simulink model "torch_xdof_sim"  (R2025b)
settings: Solver=VariableStepAuto  StartTime=0.0  StopTime=120  RelTol=1e-3
values from neighbouring files (symbols this model uses):
  framePeriod_s = 1/frameRate_hz    (= 0.005)    [setup.m]
  frameRate_hz = 200    [setup.m]
  initial_position = cur_x(1)/100    [sim_vs_flight.m]    (also in untitled2.m = -1*cur_z(1))
undefined symbols (not defined in the file or in its folder): Aircraft, magnitude
libraries: simulink x19, slpidlib x4, simulink_extras x3, uavutilslib x1, dspmathops x1
(part 1 of 2)
settings Model: Creator=amark  LastModifiedBy=aerol

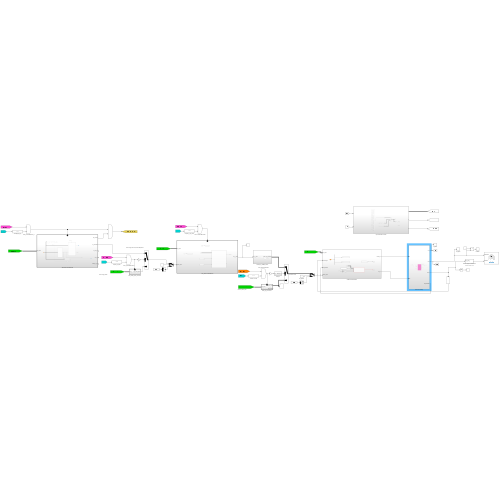
[thumbnail: Simulink's stored preview of the top-level diagram]
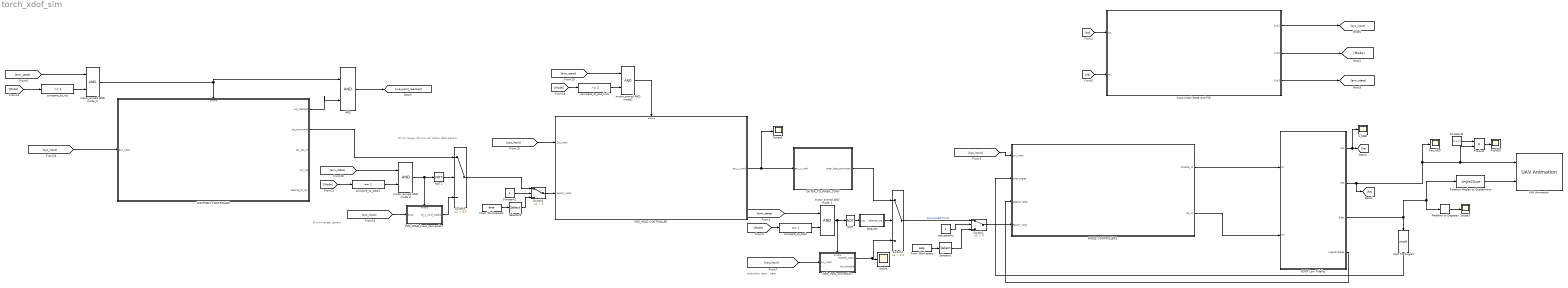
== system torch_xdof_sim ==
  note: telemetry data . para
  note: tf mini range, param
  note: tfmini range, bfs ins vel, telem data param
  6DOF Low Fidelity : Subsystem
  AND : Logic  IconShape=distinctive  AllPortsSameDT=off  OutDataTypeStr=boolean
  ANGLE CONTROLLER1 : Subsystem
  Cast To Single1 : DataTypeConversion  OutDataTypeStr=single  SaturateOnIntegerOverflow=off  RndMeth=Floor
  Constant1 : Constant
  Constant4 : Constant  Value=[1,1,-1]
  From Workspace : FromWorkspace  VariableName=data  SampleTime=0.005
  From Workspace1 : FromWorkspace  VariableName=data  OutDataTypeStr=double  SampleTime=0.005
  Input Initial State and PID : Subsystem
  NOT : Logic  Operator=NOT  IconShape=distinctive  AllPortsSameDT=off  OutDataTypeStr=boolean
  NOT1 : Logic  Operator=NOT  IconShape=distinctive  AllPortsSameDT=off  OutDataTypeStr=boolean
  OUTER_TO_INNER_CONV : Subsystem
  POS_HOLD CONTROLLER : Subsystem
  POS_HOLD_input_conversion : Subsystem
  PosNEU : Scope
      settings: ActiveDisplayYMinimum=-0.14999999999999997  ActiveDisplayYMaximum=1.3499999999999999
  Pos_NED : Scope
      settings: ActiveDisplayYMinimum=-13.68929465533385  ActiveDisplayYMaximum=21.935482841830105  DataLoggingVariableName=ScopeData7
  Product : Product
  Radians to Degrees : simulink_extras/Transformations/Radians to Degrees
  Rotation Angles to Quaternions : Angle2Quat  rotationOrder=XYZ
      settings: AttributesFormatString=Rotation Order: %<rotationOrder>
  Scope : Scope
      settings: DataLoggingVariableName=ScopeData5
  Scope1 : Scope
      settings: ActiveDisplayYMinimum=-1  ActiveDisplayYMaximum=1  DataLoggingVariableName=ScopeData8
  Scope3 : Scope
      settings: ActiveDisplayYMinimum=-18.742986936261055  ActiveDisplayYMaximum=18.74922049710748  DataLoggingVariableName=ScopeData3
  Selector1 : Selector  InputPortWidth=4  IndexOptions=Index vector (dialog)  Indices=[1 2]  OutputSizes=1
  Selector2 : Selector  InputPortWidth=4  IndexOptions=Index vector (dialog)  Indices=3  OutputSizes=1
  Stab_input_conversion : Subsystem
  Switch1 : Switch  Criteria=u2 > Threshold  SaturateOnIntegerOverflow=off  InputSameDT=off
  Switch2 : Switch  Criteria=u2 > Threshold  Threshold=0.5  SaturateOnIntegerOverflow=off  InputSameDT=off
  Switch3 : Switch  Criteria=u2 > Threshold  Threshold=0.5  SaturateOnIntegerOverflow=off  InputSameDT=off
  Switch4 : Switch  Criteria=u2 > Threshold  SaturateOnIntegerOverflow=off  InputSameDT=off
  UAV Animation : uavutilslib/UAV Animation  NumUAV=1  DynamicUAVConfig=off  UAVType=Multirotor  UAVSize=1  UAVColor=[1 0 0]  UAVTrajectoryAlpha=1  InertialZDirection=Down  RotationFormat=Quaternion  DrawMarkers=off  SampleTime=0.5
  V_NED : Scope
      settings: ActiveDisplayYMinimum=-0.14995297580074798  ActiveDisplayYMaximum=1.3495767822067306  DataLoggingVariableName=ScopeData2
  WAYPOINT CONTROLLER : Subsystem
  compare_to_pos_hold : simulink/Logic and Bit Operations/Compare To Constant  relop=>=  const=2  OutDataTypeStr=boolean
  compare_to_stab : simulink/Logic and Bit Operations/Compare To Constant  relop===  const=1  OutDataTypeStr=boolean
  compare_to_stab1 : simulink/Logic and Bit Operations/Compare To Constant  relop===  const=2  OutDataTypeStr=boolean
  compare_to_wp : simulink/Logic and Bit Operations/Compare To Constant  relop=>=  const=3  OutDataTypeStr=boolean
  delayed : Subsystem
  motor_armed AND mode 1 : Logic  IconShape=distinctive  AllPortsSameDT=off  OutDataTypeStr=boolean
  motor_armed AND mode 2 : Logic  IconShape=distinctive  AllPortsSameDT=off  OutDataTypeStr=boolean
  motor_armed AND mode2 : Logic  IconShape=distinctive  AllPortsSameDT=off  OutDataTypeStr=boolean
  motor_armed AND mode_3 : Logic  IconShape=distinctive  AllPortsSameDT=off  OutDataTypeStr=boolean
  use_params : Constant
  wires:
  ANGLE CONTROLLER1/2(roll_cc) -> 6DOF Low Fidelity/2(Mx)
  6DOF Low Fidelity/3(Euler) -> Cast To Single1/1, Rotation Angles to Quaternions/1, Radians to Degrees/1
  POS_HOLD CONTROLLER/1(acc_y_cmd) -> Scope1/1, OUTER_TO_INNER_CONV/1(acc_y_cmd)
  Cast To Single1/1 -> ANGLE CONTROLLER1/2(euler angles)
  Constant4/1 -> Product/1
  Product/1 -> PosNEU/1
  ANGLE CONTROLLER1/1(throttle_cc) -> 6DOF Low Fidelity/1(Fz)
  Rotation Angles to Quaternions/1 -> UAV Animation/2
  [Xe] -> Input Initial State and PID/1(In1)
  Input Initial State and PID/1(Out1) -> [sys_input]
  Input Initial State and PID/3(Out3) -> [arm_state]
  Input Initial State and PID/2(Out2) -> [Mode]
  [Ve] -> Input Initial State and PID/2(In2)
  6DOF Low Fidelity/2(Xe1) -> [Xe], UAV Animation/1, Product/2, Pos_NED/1
  6DOF Low Fidelity/1(Ve1) -> V_NED/1, [Ve]
  6DOF Low Fidelity/4(Angular Rates) -> ANGLE CONTROLLER1/3(angular rates)
  [sys_input] -> ANGLE CONTROLLER1/1(sys_input)
  use_params/1 -> Switch1/2
  From Workspace/1 -> Selector1/1
  Selector1/1 -> Switch1/3
  Switch1/1 -> ANGLE CONTROLLER1/4(Param_input)
  motor_armed AND mode 1/1 -> NOT/1, Stab_input_conversion/Enable
  Stab_input_conversion/1(throttle_input) -> Scope/1, Switch2/3
  NOT/1 -> delayed/1(sig)
  compare_to_stab/1 -> motor_armed AND mode 1/2
  [sys_input] -> Stab_input_conversion/1(sys_input)
  [arm_state] -> motor_armed AND mode 1/1
  [Mode] -> compare_to_stab/1
  OUTER_TO_INNER_CONV/1(inner_loop_command) -> Switch2/1
  delayed/1(delayed_sig) -> Switch2/2
  Switch2/1 -> Switch1/1  "Commanded Thrust"
  [Mode] -> compare_to_pos_hold/1
  [arm_state] -> motor_armed AND mode2/1
  motor_armed AND mode2/1 -> POS_HOLD CONTROLLER/Enable
  compare_to_pos_hold/1 -> motor_armed AND mode2/2
  motor_armed AND mode 2/1 -> NOT1/1, POS_HOLD_input_conversion/Enable
  compare_to_stab1/1 -> motor_armed AND mode 2/2
  [arm_state] -> motor_armed AND mode 2/1
  [sys_input] -> POS_HOLD_input_conversion/1(Sys1)
  [Mode] -> compare_to_stab1/1
  POS_HOLD_input_conversion/1(ve_z_cmd_input1) -> Switch3/3
  From Workspace1/1 -> Selector2/1
  NOT1/1 -> Switch3/2
  Selector2/1 -> Switch4/3
  Switch3/1 -> Switch4/1
  Constant1/1 -> Switch4/2
  Switch4/1 -> POS_HOLD CONTROLLER/2(param_input)
  [sys_input] -> POS_HOLD CONTROLLER/1(Sys_input)
  [sys_input] -> WAYPOINT CONTROLLER/1(Sys_input)
  [arm_state] -> motor_armed AND mode_3/1
  compare_to_wp/1 -> motor_armed AND mode_3/2
  [Mode] -> compare_to_wp/1
  motor_armed AND mode_3/1 -> WAYPOINT CONTROLLER/Enable, AND/1
  WAYPOINT CONTROLLER/1(wp_reached) -> AND/2
  AND/1 -> [waypoint_reached]
  WAYPOINT CONTROLLER/2(wp_command) -> Switch3/1
  Radians to Degrees/1 -> Scope3/1

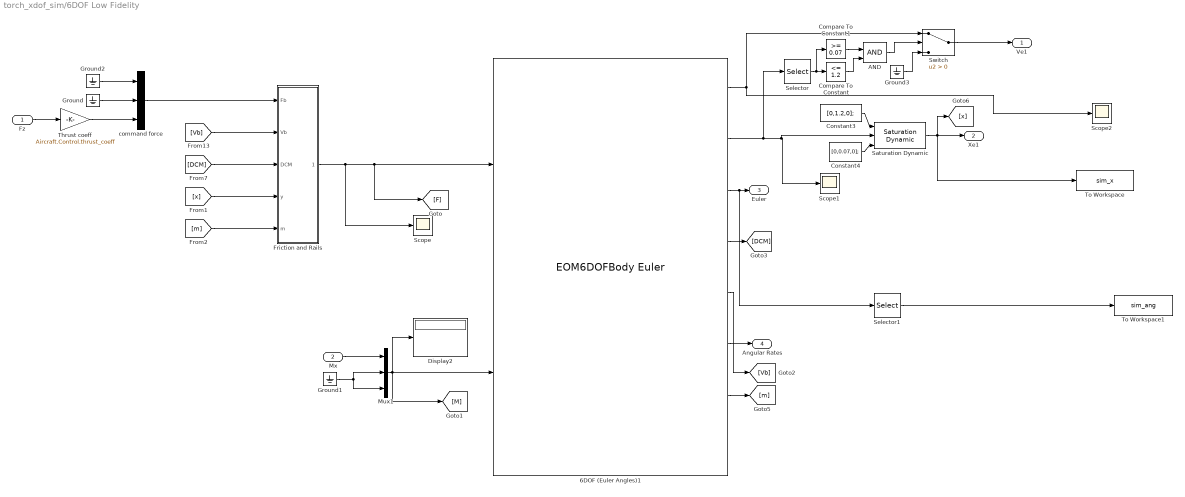
== system torch_xdof_sim/6DOF Low Fidelity ==
  Fz : Inport
  Mx : Inport  Port=2
  6DOF (Euler Angles)1 : EOM6DOFBodyEuler  xme_0=[0 initial_position 0]  mass_0=Aircraft.Mass.mass_kg  inertia=diag([3.2e-4,1e-20,1e-20])  mass_flag=on
  AND : Logic  IconShape=distinctive  AllPortsSameDT=off  OutDataTypeStr=boolean
  Compare To Constant : simulink/Logic and Bit Operations/Compare To Constant  relop=<=  const=1.2  OutDataTypeStr=boolean
  Compare To Constant1 : simulink/Logic and Bit Operations/Compare To Constant  relop=>=  const=0.07  OutDataTypeStr=boolean
  Constant3 : Constant  Value=[0,1.2,0];
  Constant4 : Constant  Value=[0,0.07,0];
  Display2 : Display
  Friction and Rails : MATLAB Function  TreatAsAtomicUnit=on
  Ground{,1..3} (4 alike) : Ground
  Mux1 : Mux  Inputs=3
  Saturation Dynamic : simulink/Discontinuities/Saturation Dynamic  OutMin=[]  OutMax=[]  OutDataTypeStr=Inherit: Same as second input  OutDataType=fixdt(1, 16)  OutScaling=2^-10  DoSatur=off
  Scope : Scope
      settings: ActiveDisplayYMinimum=-0.077435500148142641  ActiveDisplayYMaximum=0.69691950133328384  DataLoggingVariableName=ScopeData4
  Scope1 : Scope
      settings: ActiveDisplayYMinimum=-1  ActiveDisplayYMaximum=1
  Scope2 : Scope
      settings: ActiveDisplayYMinimum=-1  ActiveDisplayYMaximum=1  DataLoggingVariableName=ScopeData6
  Selector : Selector  InputPortWidth=3  IndexOptions=Index vector (dialog)  Indices=[2]  OutputSizes=1
  Selector1 : Selector  InputPortWidth=3  IndexOptions=Index vector (dialog)  Indices=1  OutputSizes=1
  Switch : Switch  Criteria=u2 > Threshold  SaturateOnIntegerOverflow=off  InputSameDT=off
  Thrust coeff : Gain  Gain=Aircraft.Control.thrust_coeff
  To Workspace : ToWorkspace  VariableName=sim_x  SaveFormat=Timeseries  SampleTime=-1
  To Workspace1 : ToWorkspace  VariableName=sim_ang  SaveFormat=Timeseries  SampleTime=-1
  command force : Mux  Inputs=3
  Ve1 : Outport
  Xe1 : Outport  Port=2
  Euler : Outport  Port=3
  Angular Rates : Outport  Port=4
  wires:
  Mux1/1 -> 6DOF (Euler Angles)1/2, [M], Display2/1
  6DOF (Euler Angles)1/3 -> Selector1/1, Euler/1
  Mx/1 -> Mux1/1
  command force/1 -> Friction and Rails/1(Fb)
  Ground1/1 -> Mux1/3, Mux1/2
  6DOF (Euler Angles)1/5 -> [Vb]
  Ground2/1 -> command force/1
  Fz/1 -> Thrust coeff/1
  6DOF (Euler Angles)1/4 -> [DCM]
  [DCM] -> Friction and Rails/3(DCM)
  [Vb] -> Friction and Rails/2(Vb)
  Ground/1 -> command force/2
  Thrust coeff/1 -> command force/3
  Friction and Rails/1(output) -> Scope/1, [F], 6DOF (Euler Angles)1/1
  [x] -> Friction and Rails/4(y)
  6DOF (Euler Angles)1/7 -> [m]
  [m] -> Friction and Rails/5(m)
  Compare To Constant1/1 -> AND/1
  Selector/1 -> Compare To Constant1/1, Compare To Constant/1
  AND/1 -> Switch/2
  Ground3/1 -> Switch/3
  Compare To Constant/1 -> AND/2
  Constant4/1 -> Saturation Dynamic/3
  Constant3/1 -> Saturation Dynamic/1
  6DOF (Euler Angles)1/2 -> Saturation Dynamic/2, Scope1/1, Selector/1
  6DOF (Euler Angles)1/1 -> Scope2/1, Switch/1
  Saturation Dynamic/1 -> To Workspace/1, Xe1/1, [x]
  Switch/1 -> Ve1/1
  6DOF (Euler Angles)1/6 -> Angular Rates/1
  Selector1/1 -> To Workspace1/1

== system torch_xdof_sim/ANGLE CONTROLLER1 ==
  sys_input : Inport
  euler angles : Inport  Port=2
  angular rates : Inport  Port=3
  Param_input : Inport  Port=4
  Demux : Demux  Outputs=3
  Demux1 : Demux  Outputs=2
  Roll Controller : Subsystem
  throttle_cc : Outport
  roll_cc : Outport  Port=2
  wires:
  Roll Controller/1(roll_cc) -> roll_cc/1  "roll_cc"
  [throttle_cc] -> throttle_cc/1  "throttle"
  euler angles/1 -> Demux/1
  Demux/1 -> Roll Controller/3(roll_angle_rad)  "roll_angle"
  angular rates/1 -> Roll Controller/4(roll_rate_radps)
  [roll_angle_cmd_rad] -> Roll Controller/2(Roll_angle_cmd_rad)  "roll_cmd"
  sys_input/1 -> Roll Controller/1(sys_input)
  Demux1/2 -> [roll_angle_cmd_rad]
  Param_input/1 -> Demux1/1
  Demux1/1 -> [throttle_cc]

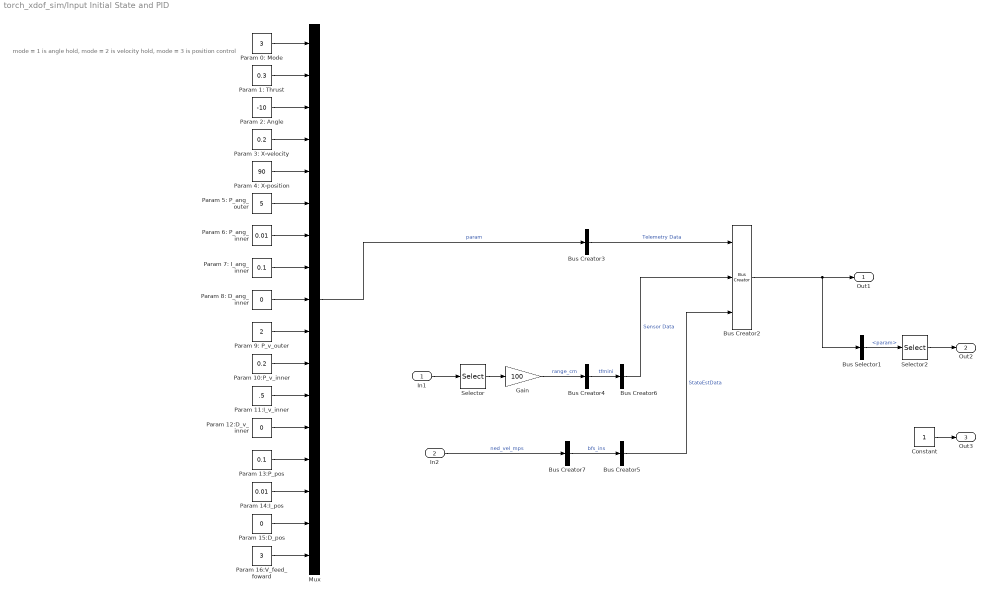
== system torch_xdof_sim/Input Initial State and PID ==
  note: mode = 1 is angle hold, mode = 2 is velocity hold, mode = 3 is position control
  In1 : Inport
  In2 : Inport  Port=2
  Bus Creator2 : BusCreator  Inputs=3
  Bus Creator{3..7} (5 alike) : BusCreator  Inputs=1
  Bus Selector1 : BusSelector  OutputSignals=Telemetry Data.param
  Constant : Constant
  Gain : Gain  Gain=100
  Mux : Mux  Inputs=17
  Param 0: Mode : Constant  Value=3
  Param 10:P_v_inner : Constant  Value=0.2
  Param 11:I_v_inner : Constant  Value=.5
  Param 12:D_v_inner : Constant  Value=0
  Param 13:P_pos : Constant  Value=0.1
  Param 14:I_pos : Constant  Value=0.01
  Param 15:D_pos : Constant  Value=0
  Param 16:V_feed_foward : Constant  Value=3
  Param 1: Thrust : Constant  Value=0.3
  Param 2: Angle : Constant  Value=-10
  Param 3: X-velocity : Constant  Value=0.2
  Param 4: X-position : Constant  Value=90
  Param 5: P_ang_outer : Constant  Value=5
  Param 6: P_ang_inner : Constant  Value=0.01
  Param 7: I_ang_inner : Constant  Value=0.1
  Param 8: D_ang_inner : Constant  Value=0
  Param 9: P_v_outer : Constant  Value=2
  Selector : Selector  InputPortWidth=3  IndexOptions=Index vector (dialog)  Indices=2  OutputSizes=1
  Selector2 : Selector  IndexMode=Zero-based  InputPortWidth=17  IndexOptions=Index vector (dialog)  Indices=0  OutputSizes=1
  Out1 : Outport
  Out2 : Outport  Port=2
  Out3 : Outport  Port=3
  wires:
  Param 3: X-velocity/1 -> Mux/4
  Bus Creator5/1 -> Bus Creator2/3  "StateEstData"
  Param 2: Angle/1 -> Mux/3
  Param 4: X-position/1 -> Mux/5
  Selector/1 -> Gain/1
  Param 11:I_v_inner/1 -> Mux/12
  Param 10:P_v_inner/1 -> Mux/11
  Param 9: P_v_outer/1 -> Mux/10
  Bus Creator6/1 -> Bus Creator2/2  "Sensor Data"
  Param 7: I_ang_inner/1 -> Mux/8
  Param 1: Thrust/1 -> Mux/2
  Param 5: P_ang_outer/1 -> Mux/6
  Bus Creator4/1 -> Bus Creator6/1  "tfmini"
  Bus Creator3/1 -> Bus Creator2/1  "Telemetry Data"
  Param 8: D_ang_inner/1 -> Mux/9
  Param 0: Mode/1 -> Mux/1
  Gain/1 -> Bus Creator4/1  "range_cm"
  Param 6: P_ang_inner/1 -> Mux/7
  In1/1 -> Selector/1
  In2/1 -> Bus Creator7/1  "ned_vel_mps"
  Bus Creator7/1 -> Bus Creator5/1  "bfs_ins"
  Bus Selector1/1 -> Selector2/1  "<param>"
  Bus Creator2/1 -> Bus Selector1/1, Out1/1
  Selector2/1 -> Out2/1
  Constant/1 -> Out3/1
  Mux/1 -> Bus Creator3/1  "param"
  Param 16:V_feed_foward/1 -> Mux/17
  Param 12:D_v_inner/1 -> Mux/13
  Param 13:P_pos/1 -> Mux/14
  Param 14:I_pos/1 -> Mux/15
  Param 15:D_pos/1 -> Mux/16

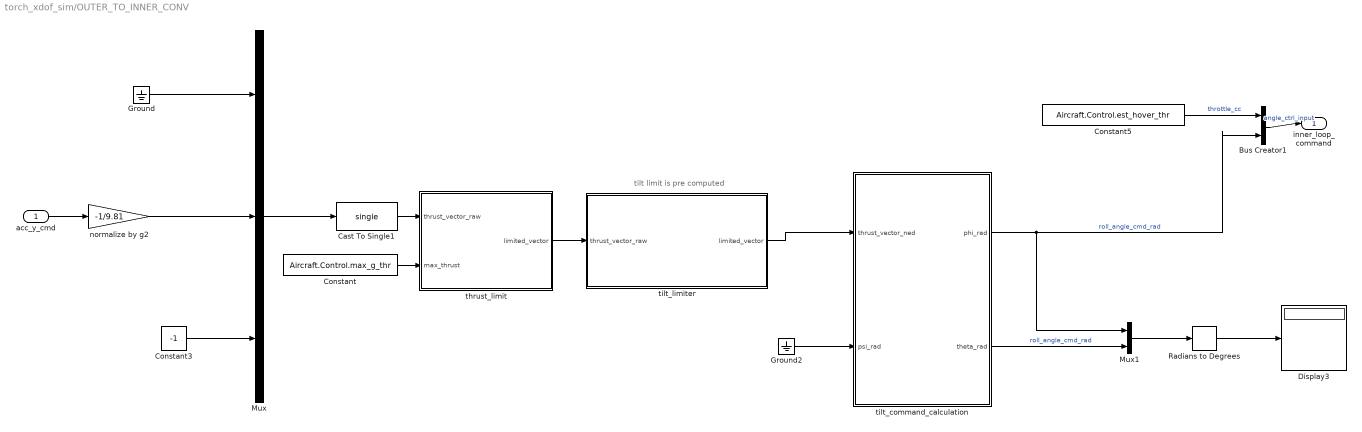
== system torch_xdof_sim/OUTER_TO_INNER_CONV ==
  note: tilt limit is pre computed
  acc_y_cmd : Inport
  " tilt_limiter" : MATLAB Function  TreatAsAtomicUnit=on
  Bus Creator1 : BusCreator  Inputs=2
  Cast To Single1 : DataTypeConversion  OutDataTypeStr=single  SaturateOnIntegerOverflow=off  RndMeth=Floor
  Constant : Constant  Value=Aircraft.Control.max_g_thr  OutDataTypeStr=single
  Constant3 : Constant  Value=-1
  Constant5 : Constant  Value=Aircraft.Control.est_hover_thr  OutDataTypeStr=single
  Display3 : Display
  Ground : Ground
  Ground2 : Ground
  Mux : Mux  Inputs=3
  Mux1 : Mux  Inputs=2
  Radians to Degrees : simulink_extras/Transformations/Radians to Degrees
  normalize by g2 : Gain  Gain=-1/9.81
  thrust_limit : MATLAB Function  TreatAsAtomicUnit=on
  tilt_command_calculation : MATLAB Function  TreatAsAtomicUnit=on
  inner_loop_command : Outport
  wires:
  Constant/1 -> thrust_limit/2(max_thrust)
  thrust_limit/1(limited_vector) -> " tilt_limiter"/1(thrust_vector_raw)
  " tilt_limiter"/1(limited_vector) -> tilt_command_calculation/1(thrust_vector_ned)
  tilt_command_calculation/1(phi_rad) -> Bus Creator1/2, Mux1/1  "roll_angle_cmd_rad"
  tilt_command_calculation/2(theta_rad) -> Mux1/2  "roll_angle_cmd_rad"
  Constant5/1 -> Bus Creator1/1  "throttle_cc"
  Ground/1 -> Mux/1
  normalize by g2/1 -> Mux/2
  Ground2/1 -> tilt_command_calculation/2(psi_rad)
  Mux/1 -> Cast To Single1/1
  Radians to Degrees/1 -> Display3/1
  Mux1/1 -> Radians to Degrees/1
  Constant3/1 -> Mux/3
  acc_y_cmd/1 -> normalize by g2/1
  Cast To Single1/1 -> thrust_limit/1(thrust_vector_raw)
  Bus Creator1/1 -> inner_loop_command/1  "angle_ctrl_input"

== system torch_xdof_sim/POS_HOLD CONTROLLER ==
  Sys_input : Inport
  param_input : Inport  Port=2
  Enable : EnablePort  StatesWhenEnabling=reset  PropagateVarSize=During execution  ShowOutputPort=on
  Horizontal speed controller : Subsystem
  acc_y_cmd : Outport
  wires:
  Horizontal speed controller/1(acc_y_cmd) -> acc_y_cmd/1  "acc_y_cmd"
  [ve_y_cmd_mps] -> Horizontal speed controller/2(ve_y_cmd_mps)
  Sys_input/1 -> Horizontal speed controller/1(sys_input)
  [pos_hold_init] -> Horizontal speed controller/3(pos_hold_init)
  Enable/1 -> [pos_hold_init]
  param_input/1 -> [ve_y_cmd_mps]

== system torch_xdof_sim/POS_HOLD_input_conversion ==
  Sys1 : Inport
  Enable : EnablePort
  Bus Selector1 : BusSelector  OutputSignals=Telemetry Data.param
  Cast1 : DataTypeConversion  OutDataTypeStr=single  SaturateOnIntegerOverflow=off  RndMeth=Floor
  Constant7 : Constant  Value=-0.3
  Constant8 : Constant  Value=0.3
  Saturation Dynamic : simulink/Discontinuities/Saturation Dynamic  OutMin=[]  OutMax=[]  OutDataTypeStr=double  OutDataType=fixdt(1, 16)  OutScaling=2^-10  DoSatur=off
  Selector : Selector  IndexMode=Zero-based  InputPortWidth=17  IndexOptions=Index vector (dialog)  Indices=3  OutputSizes=1
  ve_z_cmd_input1 : Outport
  wires:
  Sys1/1 -> Bus Selector1/1
  Constant8/1 -> Saturation Dynamic/1
  Constant7/1 -> Saturation Dynamic/3
  Bus Selector1/1 -> Selector/1  "<param>"
  Cast1/1 -> Saturation Dynamic/2
  Selector/1 -> Cast1/1
  Saturation Dynamic/1 -> ve_z_cmd_input1/1  "ve_z_cmd_mps"

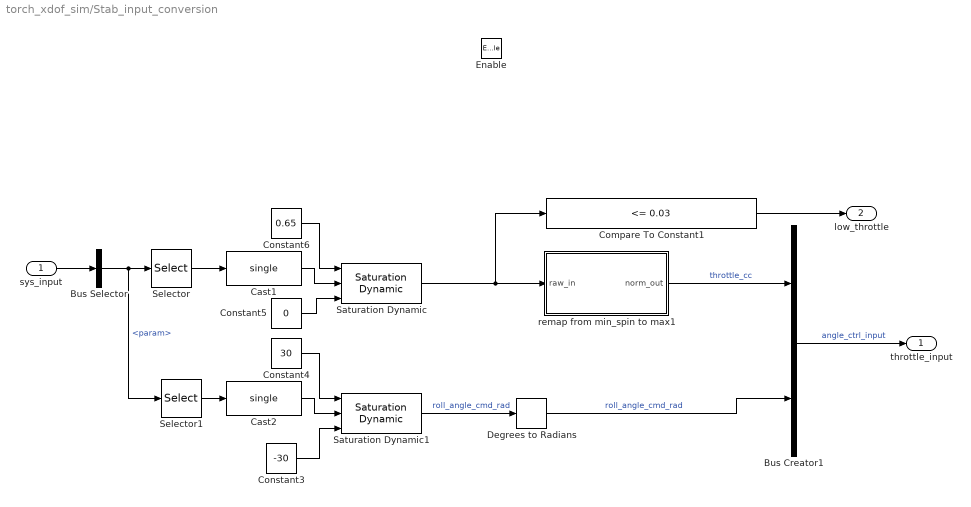
== system torch_xdof_sim/Stab_input_conversion ==
  sys_input : Inport
  Enable : EnablePort
  Bus Creator1 : BusCreator  Inputs=2
  Bus Selector : BusSelector  OutputSignals=Telemetry Data.param
  Cast1 : DataTypeConversion  OutDataTypeStr=single  SaturateOnIntegerOverflow=off  RndMeth=Floor
  Cast2 : DataTypeConversion  OutDataTypeStr=single  SaturateOnIntegerOverflow=off  RndMeth=Floor
  Compare To Constant1 : simulink/Logic and Bit Operations/Compare To Constant  relop=<=  const=0.03  OutDataTypeStr=boolean
  Constant3 : Constant  Value=-30
  Constant4 : Constant  Value=30
  Constant5 : Constant  Value=0
  Constant6 : Constant  Value=0.65
  Degrees to Radians : simulink_extras/Transformations/Degrees to Radians
  Saturation Dynamic : simulink/Discontinuities/Saturation Dynamic  OutMin=[]  OutMax=[]  OutDataTypeStr=double  OutDataType=fixdt(1, 16)  OutScaling=2^-10  DoSatur=off
  Saturation Dynamic1 : simulink/Discontinuities/Saturation Dynamic  OutMin=[]  OutMax=[]  OutDataTypeStr=single  OutDataType=fixdt(1, 16)  OutScaling=2^-10  DoSatur=off
  Selector : Selector  IndexMode=Zero-based  InputPortWidth=17  IndexOptions=Index vector (dialog)  Indices=1  OutputSizes=1
  Selector1 : Selector  IndexMode=Zero-based  InputPortWidth=17  IndexOptions=Index vector (dialog)  Indices=2  OutputSizes=1
  remap from min_spin to max1 : Subsystem
  throttle_input : Outport
  low_throttle : Outport  Port=2
  wires:
  Compare To Constant1/1 -> low_throttle/1
  Constant6/1 -> Saturation Dynamic/1
  sys_input/1 -> Bus Selector/1
  Cast1/1 -> Saturation Dynamic/2
  Selector/1 -> Cast1/1
  Constant5/1 -> Saturation Dynamic/3
  Saturation Dynamic/1 -> Compare To Constant1/1, remap from min_spin to max1/1(raw_in)
  Constant3/1 -> Saturation Dynamic1/3
  Bus Creator1/1 -> throttle_input/1  "angle_ctrl_input"
  Constant4/1 -> Saturation Dynamic1/1
  Cast2/1 -> Saturation Dynamic1/2
  Degrees to Radians/1 -> Bus Creator1/2  "roll_angle_cmd_rad"
  Saturation Dynamic1/1 -> Degrees to Radians/1  "roll_angle_cmd_rad"
  Bus Selector/1 -> Selector1/1, Selector/1  "<param>"
  Selector1/1 -> Cast2/1
  remap from min_spin to max1/1(norm_out) -> Bus Creator1/1  "throttle_cc"

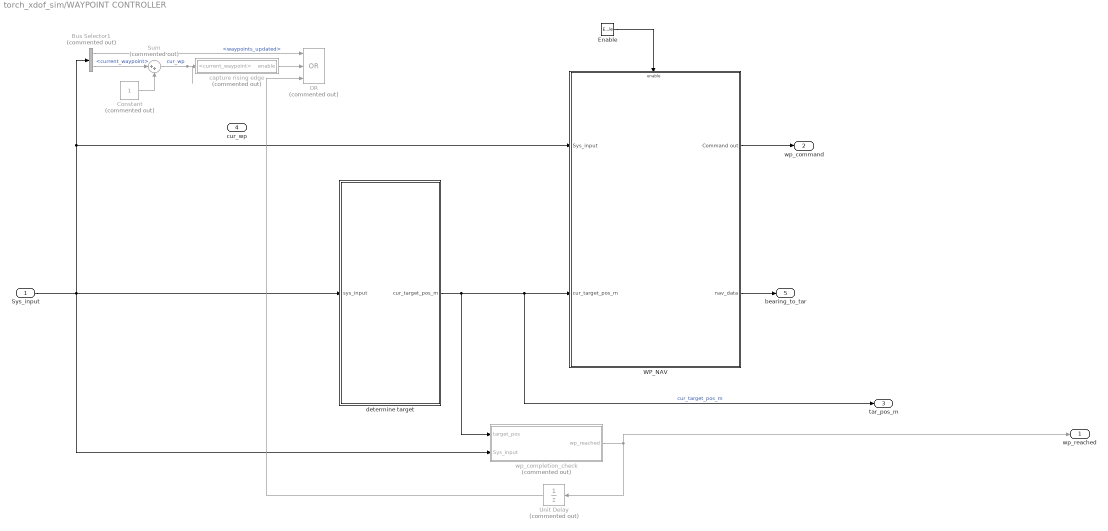
== system torch_xdof_sim/WAYPOINT CONTROLLER ==
  Sys_input : Inport
  Enable : EnablePort  StatesWhenEnabling=reset  ShowOutputPort=on
  Bus Selector1 : BusSelector  Commented=on  OutputSignals=Telemetry Data.waypoints_updated,Telemetry Data.current_waypoint
  Constant : Constant  Commented=on  OutDataTypeStr=int16
  OR : Logic  Commented=on  Operator=OR  Inputs=3  IconShape=distinctive  AllPortsSameDT=off  OutDataTypeStr=boolean
  Sum : Sum  Commented=on  Inputs=|++
  Unit Delay : UnitDelay  Commented=on  SampleTime=-1  HasFrameUpgradeWarning=on
  WP_NAV : Subsystem
  capture rising edge : Subsystem  Commented=on
  determine target : Subsystem
  wp_completion_check : Subsystem  Commented=on
  wp_reached : Outport
  wp_command : Outport  Port=2
  tar_pos_m : Outport  Port=3
  cur_wp : Outport  Port=4
  bearing_to_tar : Outport  Port=5
  wires:
  Sys_input/1 -> Bus Selector1/1, WP_NAV/1(Sys_input), wp_completion_check/2(Sys_input), determine target/1(sys_input)
  Enable/1 -> WP_NAV/Enable
  WP_NAV/1(Command out) -> wp_command/1
  determine target/1(cur_target_pos_m) -> tar_pos_m/1, WP_NAV/2(cur_target_pos_m), wp_completion_check/1(target_pos)  "cur_target_pos_m"
  Bus Selector1/1 -> OR/1  "<waypoints_updated>"
  capture rising edge/1(enable) -> OR/2
  Unit Delay/1 -> OR/3
  wp_completion_check/1(wp_reached) -> wp_reached/1, Unit Delay/1
  Constant/1 -> Sum/2
  Bus Selector1/2 -> Sum/1  "<current_waypoint>"
  Sum/1 -> capture rising edge/1(<current_waypoint>)  "cur_wp"
  WP_NAV/2(nav_data) -> bearing_to_tar/1

== system torch_xdof_sim/delayed ==
  sig : Inport
  Constant : Constant  Value=framePeriod_s  OutDataTypeStr=double
  Constant1 : Constant  Value=0.5  OutDataTypeStr=single
  Delay : Delay  DelayLengthSource=Input port
      settings: InputPortMap=u0,p1
  Divide : Product  Inputs=*/
  delayed_sig : Outport
  wires:
  Delay/1 -> delayed_sig/1
  sig/1 -> Delay/1
  Divide/1 -> Delay/2
  Constant/1 -> Divide/2
  Constant1/1 -> Divide/1

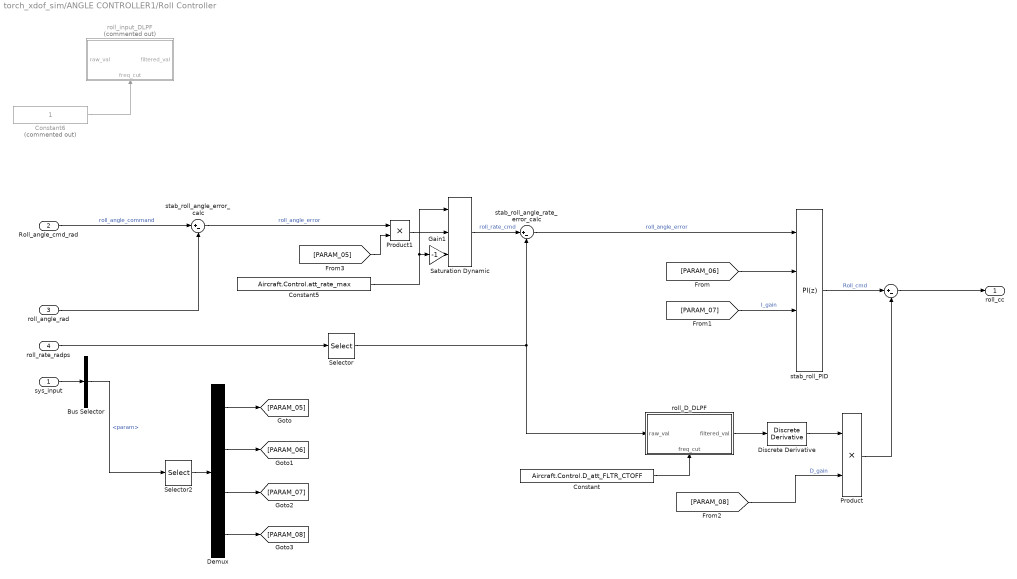
== system torch_xdof_sim/ANGLE CONTROLLER1/Roll Controller ==
  sys_input : Inport
  Roll_angle_cmd_rad : Inport  Port=2
  roll_angle_rad : Inport  Port=3
  roll_rate_radps : Inport  Port=4
  " " : Sum  Inputs=|+-
  Bus Selector : BusSelector  OutputSignals=Telemetry Data.param
  Constant : Constant  Value=Aircraft.Control.D_att_FLTR_CTOFF  OutDataTypeStr=single
  Constant5 : Constant  Value=Aircraft.Control.att_rate_max  OutDataTypeStr=single
  Constant6 : Constant  Commented=on  OutDataTypeStr=single
  Demux : Demux
  Discrete Derivative : simulink/Discrete/Discrete Derivative  gainval=1.0  ICPrevScaledInput=0.0  OutMin=[]  OutMax=[]  OutDataType=fixdt(1, 16)  OutScaling=2^-10  DoSatur=off
  Gain1 : Gain  Gain=-1
  Product : Product
  Product1 : Product
  Saturation Dynamic : simulink/Discontinuities/Saturation Dynamic  OutMin=[]  OutMax=[]  OutDataTypeStr=Inherit: Same as second input  OutDataType=fixdt(1, 16)  OutScaling=2^-10  DoSatur=off
  Selector : Selector  IndexMode=Zero-based  InputPortWidth=3  IndexOptions=Index vector (dialog)  Indices=0  OutputSizes=1
  Selector2 : Selector  IndexMode=Zero-based  InputPortWidth=17  IndexOptions=Index vector (dialog)  Indices=[5 6 7 8]  OutputSizes=1
  roll_D_DLPF : Subsystem
      settings: PortSchema="{\"entries\":[{\"content\":{\"sides\":[{\"content\":{\"connectorIds\":[\"In1\"]},\"type\":\"ConnectorPlacement.EquallySpacedRectSide\",\"uuid\":\"20236834-aeb3-4c5b-bb2e-f84447e752b5\"},{\"content\":{\"connectorIds\":[\"Out1\"],\"side\":\"RIGHT\"},\"type\":\"ConnectorPlacement.EquallySpacedRectSide\",\"uuid\":\"d668f9a1-a3df-4207-8bf1-99fb838e59b2\"},{\"content\":{\"connectorIds\":[],\"side\":\"TOP\"},\"type\":\"ConnectorPlacement.EquallySpacedRectSide\",\"uuid\":\"66cceb06-f4bc-4278-b965-2427292e46df\"},{\"content\":{\"connectorIds\":[\"In2\"],\"side\":\"BOTTOM\"},\"type\":\"ConnectorPlacement.EquallySpacedRectSide\",\"uuid\":\"8fdaac6a-cb03-4bd4-87bb-7bafd10bc297\"}]},\"type\":\"ConnectorPlacement.EquallySpacedConnector\",\"uuid\":\"3dc29a9a-e794-478d-b7df-452e6c2d3f66\"}],\"packageUris\":[\"http://schema.mathworks.com/mf0/Connector/R2020b\"],\"version\":\"1.0\"}"
  roll_input_DLPF : Subsystem  Commented=on
      settings: PortSchema="{\"entries\":[{\"content\":{\"sides\":[{\"content\":{\"connectorIds\":[\"In1\"]},\"type\":\"ConnectorPlacement.EquallySpacedRectSide\",\"uuid\":\"20236834-aeb3-4c5b-bb2e-f84447e752b5\"},{\"content\":{\"connectorIds\":[\"Out1\"],\"side\":\"RIGHT\"},\"type\":\"ConnectorPlacement.EquallySpacedRectSide\",\"uuid\":\"d668f9a1-a3df-4207-8bf1-99fb838e59b2\"},{\"content\":{\"connectorIds\":[],\"side\":\"TOP\"},\"type\":\"ConnectorPlacement.EquallySpacedRectSide\",\"uuid\":\"66cceb06-f4bc-4278-b965-2427292e46df\"},{\"content\":{\"connectorIds\":[\"In2\"],\"side\":\"BOTTOM\"},\"type\":\"ConnectorPlacement.EquallySpacedRectSide\",\"uuid\":\"8fdaac6a-cb03-4bd4-87bb-7bafd10bc297\"}]},\"type\":\"ConnectorPlacement.EquallySpacedConnector\",\"uuid\":\"3dc29a9a-e794-478d-b7df-452e6c2d3f66\"}],\"packageUris\":[\"http://schema.mathworks.com/mf0/Connector/R2020b\"],\"version\":\"1.0\"}"
  stab_roll_PID : slpidlib/PID Controller  Controller=PI  Form=Parallel  TimeDomain=Discrete-time  UseExternalTs=off  SampleTime=framePeriod_s  IntegratorMethod=Forward Euler  FilterMethod=Forward Euler  ControllerParametersSource=external  P=0.335  I=0.005  UseKiTs=off  D=0  UseExternalDerivativeSource=off  N=100  UseFilter=off  TunerSelectOption=Transfer Function Based (PID Tuner App)  InitialConditionSource=internal  InitialConditionForIntegrator=0  InitialConditionForFilter=0  DifferentiatorICPrevScaledInput=0  ExternalReset=either  TrackingMode=off  Kt=1  LimitOutput=on  SatLimitsSource=internal  UpperSaturationLimit=100  LowerSaturationLimit=-100  LinearizeAsGain=on  AntiWindupMode=clamping  Kb=1  LimitIntegrator=off  UpperIntegratorSaturationLimit=inf  LowerIntegratorSaturationLimit=-inf  POutMin=[]  POutMax=[]  IOutMin=[]  IOutMax=[]  DOutMin=[]  DOutMax=[]  NOutMin=[]  NOutMax=[]  SumOutMin=[]  SumOutMax=[]  SaturationOutMin=[]  SaturationOutMax=[]  PParamMin=[]  PParamMax=[]  IParamMin=[]  IParamMax=[]  DParamMin=[]  DParamMax=[]  NParamMin=[]  NParamMax=[]  KbParamMin=[]  KbParamMax=[]  KtParamMin=[]  KtParamMax=[]  KbOutMin=[]  KbOutMax=[]  KtOutMin=[]  KtOutMax=[]  IntegratorOutMin=[]  IntegratorOutMax=[]  FilterOutMin=[]  FilterOutMax=[]  SumI1OutMin=[]  SumI1OutMax=[]  SumI2OutMin=[]  SumI2OutMax=[]  SumI3OutMin=[]  SumI3OutMax=[]  SumI4OutMin=[]  SumI4OutMax=[]  SumDOutMin=[]  SumDOutMax=[]  DifferentiatorOutMin=[]  DifferentiatorOutMax=[]  FilterDiffOutCoefMin=[]  FilterDiffOutCoefMax=[]  ReciprocalOutMin=[]  ReciprocalOutMax=[]  SumDenOutMin=[]  SumDenOutMax=[]  SumNumOutMin=[]  SumNumOutMax=[]  DivideOutMin=[]  DivideOutMax=[]  UdiffTsProdOutMin=[]  UdiffTsProdOutMax=[]  NTsProdOutMin=[]  NTsProdOutMax=[]  UintegralTsProdOutMin=[]  UintegralTsProdOutMax=[]  UngainTsProdOutMin=[]  UngainTsProdOutMax=[]  ClampingZeroOutDataTypeStr=Inherit: Inherit via back propagation  ClampingZeroOutMin=[]  ClampingZeroOutMax=[]  FilterDenConstantOutDataTypeStr=Inherit: Inherit via back propagation  FilterDenConstantOutMin=[]  FilterDenConstantOutMax=[]  PCopyOutDataTypeStr=Inherit: Inherit via back propagation  PCopyOutMin=[]  PCopyOutMax=[]  NCopyOutDataTypeStr=Inherit: Inherit via back propagation  NCopyOutMin=[]  NCopyOutMax=[]  IntegratorContinuousStateAttributes=''  IntegratorStateMustResolveToSignalObject=off  IntegratorRTWStateStorageClass=Auto  FilterContinuousStateAttributes=''  FilterStateMustResolveToSignalObject=off  FilterRTWStateStorageClass=Auto  ParallelPVariant=ExternalParameters  IdealPVariant=Disabled  IVariant=ExternalParameters  DVariant=Disabled  IntegratorVariant=Discrete  SatVariant=Enabled  AWVariant=DiscClampingParallel  PCopyVariant=Disabled  TRVariant=Disabled  FdbkBlocksVariant=Forward  IdealPFdbkVariant=Disabled  SatFdbkVariant=Disabled  DerivativeFilterVariant=Disabled  NVariant=Disabled  NCopyVariant=Disabled_SignalSpec  FilterICVariant=Disabled  IntegratorICVariant=InternalICs  ExternalResetVariant=ExternalReset  TRSumVariant=Passthrough  SumFdbkVariant=Disabled  SumVariant=Sum_PI  TsampFilterVariant=InternalTs  TsampNgainVariant=Passthrough  TsampIntegralVariant=Disabled_SignalSpec  ExternalSaturationOutDataTypeStr=Inherit: Same as second input  DerivativeSourceVariant=Disabled  PreIntVariant=InternalPreInt
  stab_roll_angle_error_calc : Sum  Inputs=|+-
  stab_roll_angle_rate_error_calc : Sum  Inputs=|+-
  roll_cc : Outport
  wires:
  " "/1 -> roll_cc/1
  roll_rate_radps/1 -> Selector/1
  [PARAM_06] -> stab_roll_PID/2
  [PARAM_07] -> stab_roll_PID/3  "I_gain"
  [PARAM_08] -> Product/2  "D_gain"
  Constant5/1 -> Gain1/1, Saturation Dynamic/1
  Gain1/1 -> Saturation Dynamic/3
  Product1/1 -> Saturation Dynamic/2
  stab_roll_angle_error_calc/1 -> Product1/1  "roll_angle_error"
  [PARAM_05] -> Product1/2
  Discrete Derivative/1 -> Product/1
  Constant/1 -> roll_D_DLPF/2(freq_cut)
  roll_D_DLPF/1(filtered_val) -> Discrete Derivative/1
  stab_roll_angle_rate_error_calc/1 -> stab_roll_PID/1  "roll_angle_error"
  stab_roll_PID/1 -> " "/1  "Roll_cmd"
  Product/1 -> " "/2
  Constant6/1 -> roll_input_DLPF/2(freq_cut)
  Roll_angle_cmd_rad/1 -> stab_roll_angle_error_calc/1  "roll_angle_command"
  Selector/1 -> stab_roll_angle_rate_error_calc/2, roll_D_DLPF/1(raw_val)
  Saturation Dynamic/1 -> stab_roll_angle_rate_error_calc/1  "roll_rate_cmd"
  roll_angle_rad/1 -> stab_roll_angle_error_calc/2
  Demux/1 -> [PARAM_05]
  Demux/4 -> [PARAM_08]
  Bus Selector/1 -> Selector2/1  "<param>"
  Selector2/1 -> Demux/1
  Demux/2 -> [PARAM_06]
  Demux/3 -> [PARAM_07]
  sys_input/1 -> Bus Selector/1

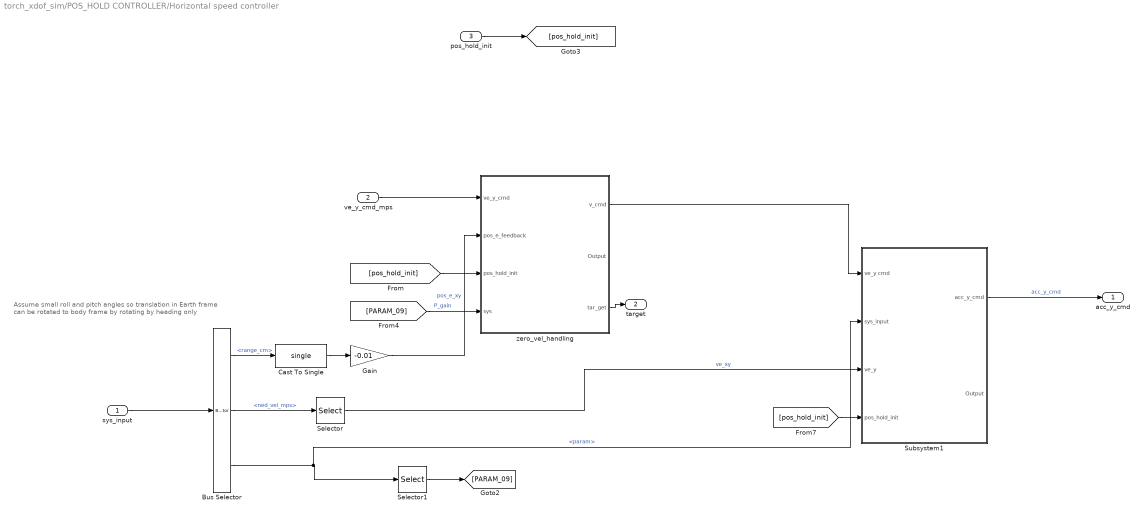
== system torch_xdof_sim/POS_HOLD CONTROLLER/Horizontal speed controller ==
  note: Assume small roll and pitch angles so translation in Earth frame can be rotated to body frame by rotating by heading only
  sys_input : Inport
  ve_y_cmd_mps : Inport  Port=2
  pos_hold_init : Inport  Port=3
  Bus Selector : BusSelector  OutputSignals=Sensor Data.tfmini.range_cm,StateEstData.bfs_ins.ned_vel_mps,Telemetry Data.param
  Cast To Single : DataTypeConversion  OutDataTypeStr=single  SaturateOnIntegerOverflow=off  RndMeth=Floor
  Gain : Gain  Gain=-0.01
  Selector : Selector  InputPortWidth=3  IndexOptions=Index vector (dialog)  Indices=2  OutputSizes=1
  Selector1 : Selector  IndexMode=Zero-based  InputPortWidth=17  IndexOptions=Index vector (dialog)  Indices=9  OutputSizes=1
  Subsystem1 : Subsystem
  zero_vel_handling : Subsystem
  acc_y_cmd : Outport
  target : Outport  Port=2
  wires:
  Subsystem1/1(acc_y_cmd) -> acc_y_cmd/1  "acc_y_cmd"
  sys_input/1 -> Bus Selector/1
  pos_hold_init/1 -> [pos_hold_init]
  [pos_hold_init] -> Subsystem1/4(pos_hold_init)
  Bus Selector/2 -> Selector/1  "<ned_vel_mps>"
  ve_y_cmd_mps/1 -> zero_vel_handling/1(ve_y_cmd)
  [pos_hold_init] -> zero_vel_handling/3(pos_hold_init)
  zero_vel_handling/1(v_cmd) -> Subsystem1/1(ve_y cmd)
  Selector/1 -> Subsystem1/3(ve_y)  "ve_xy"
  zero_vel_handling/3(tar_get) -> target/1
  [PARAM_09] -> zero_vel_handling/4(sys)  "P_gain"
  Bus Selector/1 -> Cast To Single/1  "<range_cm>"
  Cast To Single/1 -> Gain/1
  Gain/1 -> zero_vel_handling/2(pos_e_feedback)  "pos_e_xy"
  Selector1/1 -> [PARAM_09]
  Bus Selector/3 -> Subsystem1/2(sys_input), Selector1/1  "<param>"

== system torch_xdof_sim/Stab_input_conversion/remap from min_spin to max1 ==
  raw_in : Inport
  Constant4 : Constant  Value=0  OutDataTypeStr=single
  Constant5 : Constant  Value=Aircraft.Control.motor_spin_min  OutDataTypeStr=double
  Constant6 : Constant  Value=0.8  OutDataTypeStr=double
  Constant7 : Constant  OutDataTypeStr=single
  remap1 : MATLAB Function  TreatAsAtomicUnit=on
  norm_out : Outport
  wires:
  Constant6/1 -> remap1/5(out_max)
  Constant5/1 -> remap1/4(out_min)
  remap1/1(norm_out) -> norm_out/1
  Constant4/1 -> remap1/2(in_min)
  Constant7/1 -> remap1/3(in_max)
  raw_in/1 -> remap1/1(raw_in)

== system torch_xdof_sim/WAYPOINT CONTROLLER/WP_NAV ==
  Sys_input : Inport
  cur_target_pos_m : Inport  Port=2
  Enable : EnablePort
  Horizontal position controller : Subsystem
  Command out : Outport
  nav_data : Outport  Port=2
  wires:
  Horizontal position controller/1(ve_y_cmd_mps) -> Command out/1  "ve_y_cmd_mps"
  Sys_input/1 -> Horizontal position controller/1(Sys_input)
  cur_target_pos_m/1 -> Horizontal position controller/2(cur_target_pos_m)
  Horizontal position controller/2(nav_data) -> nav_data/1

== system torch_xdof_sim/WAYPOINT CONTROLLER/capture rising edge ==
  <current_waypoint> : Inport
  Detect Change1 : simulink/Logic and Bit Operations/Detect Change  vinit=-1  OutDataTypeStr=boolean
  Detect Rise Positive : simulink/Logic and Bit Operations/Detect Rise Positive  Commented=through  vinit=0  OutDataTypeStr=boolean
  enable : Outport
  wires:
  <current_waypoint>/1 -> Detect Change1/1
  Detect Rise Positive/1 -> enable/1
  Detect Change1/1 -> Detect Rise Positive/1

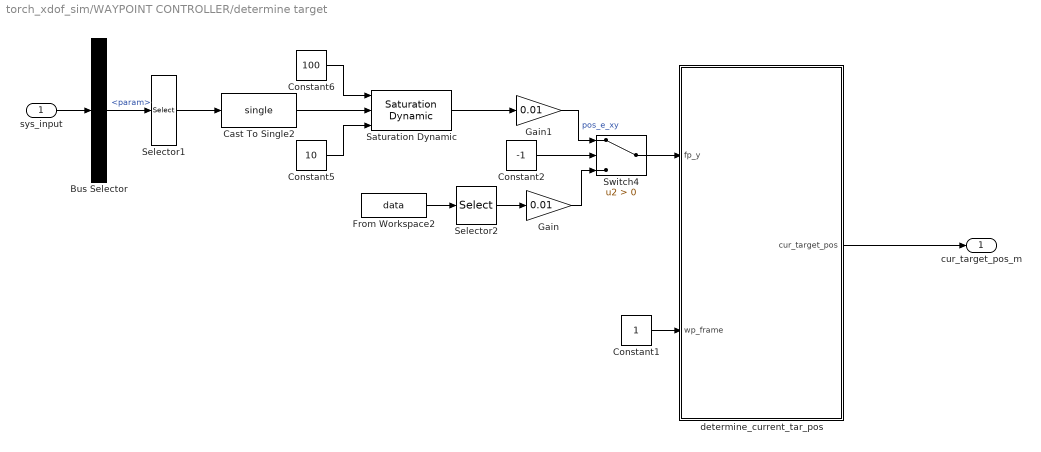
== system torch_xdof_sim/WAYPOINT CONTROLLER/determine target ==
  sys_input : Inport
  Bus Selector : BusSelector  OutputSignals=Telemetry Data.param
  Cast To Single2 : DataTypeConversion  OutDataTypeStr=single  SaturateOnIntegerOverflow=off  RndMeth=Floor
  Constant1 : Constant  OutDataTypeStr=uint8
  Constant2 : Constant  Value=-1
  Constant5 : Constant  Value=10
  Constant6 : Constant  Value=100
  From Workspace2 : FromWorkspace  VariableName=data  SampleTime=0.005
  Gain : Gain  Gain=0.01
  Gain1 : Gain  Gain=0.01
  Saturation Dynamic : simulink/Discontinuities/Saturation Dynamic  OutMin=[]  OutMax=[]  OutDataTypeStr=double  OutDataType=fixdt(1, 16)  OutScaling=2^-10  DoSatur=off
  Selector1 : Selector  IndexMode=Zero-based  InputPortWidth=17  IndexOptions=Index vector (dialog)  Indices=4  OutputSizes=1
  Selector2 : Selector  InputPortWidth=4  IndexOptions=Index vector (dialog)  Indices=4  OutputSizes=1
  Switch4 : Switch  Criteria=u2 > Threshold  SaturateOnIntegerOverflow=off  InputSameDT=off
  determine_current_tar_pos : MATLAB Function  TreatAsAtomicUnit=on
  cur_target_pos_m : Outport
  wires:
  sys_input/1 -> Bus Selector/1
  Constant1/1 -> determine_current_tar_pos/2(wp_frame)
  determine_current_tar_pos/1(cur_target_pos) -> cur_target_pos_m/1
  Bus Selector/1 -> Selector1/1  "<param>"
  Cast To Single2/1 -> Saturation Dynamic/2
  Constant5/1 -> Saturation Dynamic/3
  Constant6/1 -> Saturation Dynamic/1
  Selector1/1 -> Cast To Single2/1
  Saturation Dynamic/1 -> Gain1/1
  Gain1/1 -> Switch4/1  "pos_e_xy"
  Gain/1 -> Switch4/3
  Constant2/1 -> Switch4/2
  Selector2/1 -> Gain/1
  From Workspace2/1 -> Selector2/1
  Switch4/1 -> determine_current_tar_pos/1(fp_y)

== system torch_xdof_sim/WAYPOINT CONTROLLER/wp_completion_check ==
  note: Output wp_reached cmd only when distance between current pos and target pos is less than wp_radius.
  target_pos : Inport
  Sys_input : Inport  Port=2
  Bus Selector : BusSelector  OutputSignals=StateEstData.aux_ins.ned_pos_m
  Constant : Constant  Value=Aircraft.Control.wp_radius  OutDataTypeStr=single
  check_wp_reached : MATLAB Function  TreatAsAtomicUnit=on
  wp_reached : Outport
  wires:
  Sys_input/1 -> Bus Selector/1
  Bus Selector/1 -> check_wp_reached/2(ned_pos)  "<ned_pos_m>"
  check_wp_reached/1(reached) -> wp_reached/1
  target_pos/1 -> check_wp_reached/1(target_pos)
  Constant/1 -> check_wp_reached/3(Aircraft_Control_wp_radius)

== system torch_xdof_sim/ANGLE CONTROLLER1/Roll Controller/roll_D_DLPF ==
  raw_val : Inport
  freq_cut : Inport  Port=2
  Cast To Single : DataTypeConversion  OutDataTypeStr=single  SaturateOnIntegerOverflow=off  RndMeth=Floor
  Constant : Constant  Value=frameRate_hz  OutDataTypeStr=single
  MATLAB Function : MATLAB Function  TreatAsAtomicUnit=on
  Unit Delay : UnitDelay  SampleTime=-1  HasFrameUpgradeWarning=on
  filtered_val : Outport
  wires:
  freq_cut/1 -> MATLAB Function/3(freq_cut)
  MATLAB Function/1(filtered_val) -> Unit Delay/1, filtered_val/1
  Unit Delay/1 -> Cast To Single/1
  raw_val/1 -> MATLAB Function/2(raw_val)
  Constant/1 -> MATLAB Function/4(samp_freq)
  Cast To Single/1 -> MATLAB Function/1(prev_val)

== system torch_xdof_sim/ANGLE CONTROLLER1/Roll Controller/roll_input_DLPF ==
  raw_val : Inport
  freq_cut : Inport  Port=2
  Constant : Constant  Value=frameRate_hz  OutDataTypeStr=single
  MATLAB Function : MATLAB Function  TreatAsAtomicUnit=on
  Unit Delay : UnitDelay  SampleTime=-1  HasFrameUpgradeWarning=on
  filtered_val : Outport
  wires:
  Constant/1 -> MATLAB Function/4(samp_freq)
  raw_val/1 -> MATLAB Function/2(raw_val)
  Unit Delay/1 -> MATLAB Function/1(prev_val)
  MATLAB Function/1(filtered_val) -> filtered_val/1, Unit Delay/1
  freq_cut/1 -> MATLAB Function/3(freq_cut)

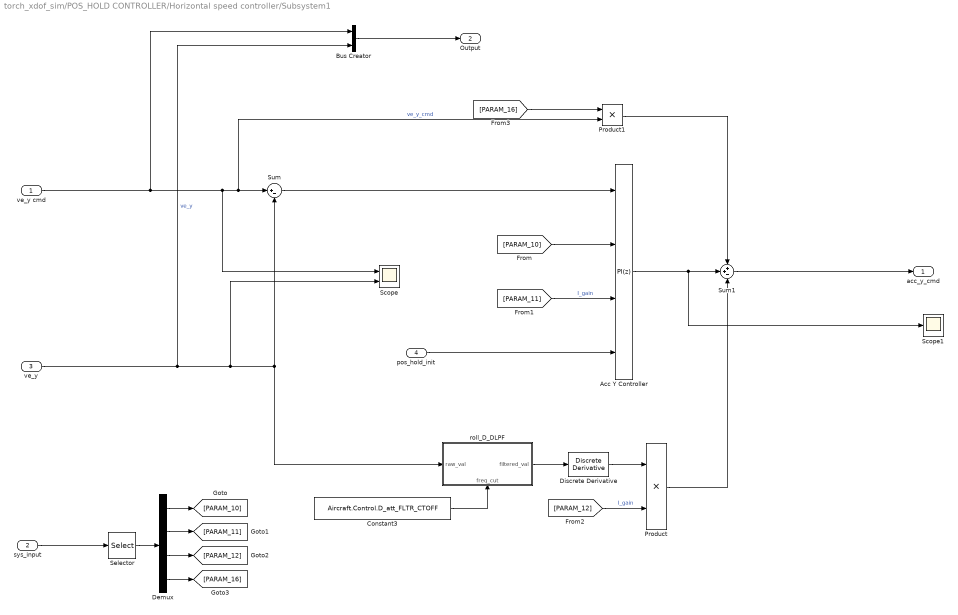
== system torch_xdof_sim/POS_HOLD CONTROLLER/Horizontal speed controller/Subsystem1 ==
  ve_y cmd : Inport
  sys_input : Inport  Port=2
  ve_y : Inport  Port=3
  pos_hold_init : Inport  Port=4
  Acc Y Controller : slpidlib/PID Controller  Controller=PI  Form=Parallel  TimeDomain=Discrete-time  UseExternalTs=off  SampleTime=framePeriod_s  IntegratorMethod=Forward Euler  FilterMethod=Forward Euler  ControllerParametersSource=external  P=0.335  I=0.005  UseKiTs=off  D=0  UseExternalDerivativeSource=off  N=100  UseFilter=off  TunerSelectOption=Transfer Function Based (PID Tuner App)  InitialConditionSource=internal  InitialConditionForIntegrator=0  InitialConditionForFilter=0  DifferentiatorICPrevScaledInput=0  ExternalReset=either  TrackingMode=off  Kt=1  LimitOutput=off  SatLimitsSource=internal  UpperSaturationLimit=Aircraft.Control.roll_angle_lim  LowerSaturationLimit=-Aircraft.Control.roll_angle_lim  LinearizeAsGain=off  AntiWindupMode=clamping  Kb=1  LimitIntegrator=off  UpperIntegratorSaturationLimit=inf  LowerIntegratorSaturationLimit=-inf  POutMin=[]  POutMax=[]  IOutMin=[]  IOutMax=[]  DOutMin=[]  DOutMax=[]  NOutMin=[]  NOutMax=[]  SumOutMin=[]  SumOutMax=[]  SaturationOutMin=[]  SaturationOutMax=[]  PParamMin=[]  PParamMax=[]  IParamMin=[]  IParamMax=[]  DParamMin=[]  DParamMax=[]  NParamMin=[]  NParamMax=[]  KbParamMin=[]  KbParamMax=[]  KtParamMin=[]  KtParamMax=[]  KbOutMin=[]  KbOutMax=[]  KtOutMin=[]  KtOutMax=[]  IntegratorOutMin=[]  IntegratorOutMax=[]  FilterOutMin=[]  FilterOutMax=[]  SumI1OutMin=[]  SumI1OutMax=[]  SumI2OutMin=[]  SumI2OutMax=[]  SumI3OutMin=[]  SumI3OutMax=[]  SumI4OutMin=[]  SumI4OutMax=[]  SumDOutMin=[]  SumDOutMax=[]  DifferentiatorOutMin=[]  DifferentiatorOutMax=[]  FilterDiffOutCoefMin=[]  FilterDiffOutCoefMax=[]  ReciprocalOutMin=[]  ReciprocalOutMax=[]  SumDenOutMin=[]  SumDenOutMax=[]  SumNumOutMin=[]  SumNumOutMax=[]  DivideOutMin=[]  DivideOutMax=[]  UdiffTsProdOutMin=[]  UdiffTsProdOutMax=[]  NTsProdOutMin=[]  NTsProdOutMax=[]  UintegralTsProdOutMin=[]  UintegralTsProdOutMax=[]  UngainTsProdOutMin=[]  UngainTsProdOutMax=[]  ClampingZeroOutDataTypeStr=Inherit: Inherit via back propagation  ClampingZeroOutMin=[]  ClampingZeroOutMax=[]  FilterDenConstantOutDataTypeStr=Inherit: Inherit via back propagation  FilterDenConstantOutMin=[]  FilterDenConstantOutMax=[]  PCopyOutDataTypeStr=Inherit: Inherit via back propagation  PCopyOutMin=[]  PCopyOutMax=[]  NCopyOutDataTypeStr=Inherit: Inherit via back propagation  NCopyOutMin=[]  NCopyOutMax=[]  IntegratorContinuousStateAttributes=''  IntegratorStateMustResolveToSignalObject=off  IntegratorRTWStateStorageClass=Auto  FilterContinuousStateAttributes=''  FilterStateMustResolveToSignalObject=off  FilterRTWStateStorageClass=Auto  ParallelPVariant=ExternalParameters  IdealPVariant=Disabled  IVariant=ExternalParameters  DVariant=Disabled  IntegratorVariant=Discrete  SatVariant=Disabled  AWVariant=Passthrough  PCopyVariant=Disabled  TRVariant=Disabled  FdbkBlocksVariant=Forward  IdealPFdbkVariant=Disabled  SatFdbkVariant=Disabled  DerivativeFilterVariant=Disabled  NVariant=Disabled  NCopyVariant=Disabled_SignalSpec  FilterICVariant=Disabled  IntegratorICVariant=InternalICs  ExternalResetVariant=ExternalReset  TRSumVariant=Passthrough  SumFdbkVariant=Disabled  SumVariant=Sum_PI  TsampFilterVariant=InternalTs  TsampNgainVariant=Passthrough  TsampIntegralVariant=Disabled_SignalSpec  ExternalSaturationOutDataTypeStr=Inherit: Same as second input  DerivativeSourceVariant=Disabled  PreIntVariant=InternalPreInt
  Bus Creator : BusCreator  Inputs=2
  Constant3 : Constant  Value=Aircraft.Control.D_att_FLTR_CTOFF  OutDataTypeStr=single
  Demux : Demux
  Discrete Derivative : simulink/Discrete/Discrete Derivative  gainval=1.0  ICPrevScaledInput=0.0  OutMin=[]  OutMax=[]  OutDataType=fixdt(1, 16)  OutScaling=2^-10  DoSatur=off
  Product : Product
  Product1 : Product
  Scope : Scope  NumInputPorts=2
      settings: ActiveDisplayYMinimum=-1  ActiveDisplayYMaximum=1  DataLoggingVariableName=ScopeData9
  Scope1 : Scope
      settings: ActiveDisplayYMinimum=-1  ActiveDisplayYMaximum=1  DataLoggingVariableName=ScopeData10
  Selector : Selector  IndexMode=Zero-based  InputPortWidth=17  IndexOptions=Index vector (dialog)  Indices=[10 11 12 16]  OutputSizes=1
  Sum : Sum  Inputs=|+-
  Sum1 : Sum  Inputs=++-
  roll_D_DLPF : Subsystem
      settings: PortSchema="{\"entries\":[{\"content\":{\"sides\":[{\"content\":{\"connectorIds\":[\"In1\"]},\"type\":\"ConnectorPlacement.EquallySpacedRectSide\",\"uuid\":\"20236834-aeb3-4c5b-bb2e-f84447e752b5\"},{\"content\":{\"connectorIds\":[\"Out1\"],\"side\":\"RIGHT\"},\"type\":\"ConnectorPlacement.EquallySpacedRectSide\",\"uuid\":\"d668f9a1-a3df-4207-8bf1-99fb838e59b2\"},{\"content\":{\"connectorIds\":[],\"side\":\"TOP\"},\"type\":\"ConnectorPlacement.EquallySpacedRectSide\",\"uuid\":\"66cceb06-f4bc-4278-b965-2427292e46df\"},{\"content\":{\"connectorIds\":[\"In2\"],\"side\":\"BOTTOM\"},\"type\":\"ConnectorPlacement.EquallySpacedRectSide\",\"uuid\":\"8fdaac6a-cb03-4bd4-87bb-7bafd10bc297\"}]},\"type\":\"ConnectorPlacement.EquallySpacedConnector\",\"uuid\":\"3dc29a9a-e794-478d-b7df-452e6c2d3f66\"}],\"packageUris\":[\"http://schema.mathworks.com/mf0/Connector/R2020b\"],\"version\":\"1.0\"}"
  acc_y_cmd : Outport
  Output : Outport  Port=2
  wires:
  ve_y/1 -> Bus Creator/2, Scope/2, roll_D_DLPF/1(raw_val), Sum/2  "ve_y"
  Sum/1 -> Acc Y Controller/1
  Sum1/1 -> acc_y_cmd/1
  [PARAM_10] -> Acc Y Controller/2
  [PARAM_11] -> Acc Y Controller/3  "I_gain"
  pos_hold_init/1 -> Acc Y Controller/4
  Discrete Derivative/1 -> Product/1
  Constant3/1 -> roll_D_DLPF/2(freq_cut)
  roll_D_DLPF/1(filtered_val) -> Discrete Derivative/1
  Bus Creator/1 -> Output/1
  ve_y cmd/1 -> Scope/1, Product1/2, Sum/1, Bus Creator/1  "ve_y_cmd"
  [PARAM_12] -> Product/2  "I_gain"
  Demux/1 -> [PARAM_10]
  Selector/1 -> Demux/1
  sys_input/1 -> Selector/1
  Demux/3 -> [PARAM_12]
  Demux/2 -> [PARAM_11]
  [PARAM_16] -> Product1/1
  Acc Y Controller/1 -> Scope1/1, Sum1/2
  Product/1 -> Sum1/3
  Product1/1 -> Sum1/1
  Demux/4 -> [PARAM_16]

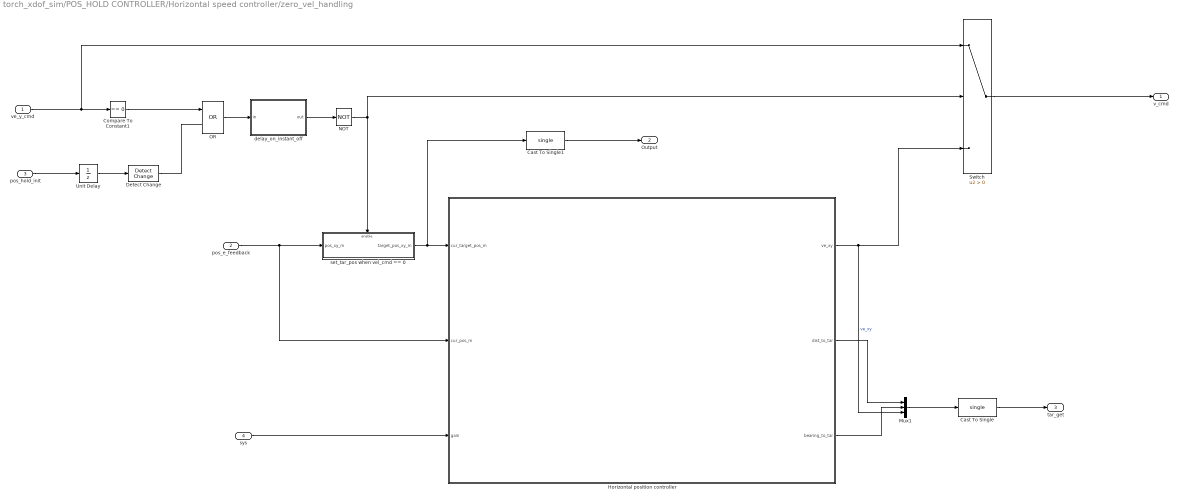
== system torch_xdof_sim/POS_HOLD CONTROLLER/Horizontal speed controller/zero_vel_handling ==
  ve_y_cmd : Inport
  pos_e_feedback : Inport  Port=2
  pos_hold_init : Inport  Port=3
  sys : Inport  Port=4
  Cast To Single : DataTypeConversion  OutDataTypeStr=single  SaturateOnIntegerOverflow=off  RndMeth=Floor
  Cast To Single1 : DataTypeConversion  OutDataTypeStr=single  SaturateOnIntegerOverflow=off  RndMeth=Floor
  Compare To Constant1 : simulink/Logic and Bit Operations/Compare To Constant  relop===  const=0  OutDataTypeStr=boolean
  Detect Change : simulink/Logic and Bit Operations/Detect Change  vinit=0  OutDataTypeStr=boolean
  Horizontal position controller : Subsystem
  Mux1 : Mux  Inputs=3
  NOT : Logic  Operator=NOT  IconShape=distinctive  AllPortsSameDT=off  OutDataTypeStr=boolean
  OR : Logic  Operator=OR  IconShape=distinctive  AllPortsSameDT=off  OutDataTypeStr=boolean
  Switch : Switch  Criteria=u2 > Threshold  SaturateOnIntegerOverflow=off  InputSameDT=off
  Unit Delay : UnitDelay  SampleTime=-1  HasFrameUpgradeWarning=on
  delay_on_instant_off : Subsystem
  set_tar_pos when vel_cmd == 0 : Subsystem  TreatAsAtomicUnit=on
  v_cmd : Outport
  Output : Outport  Port=2
  tar_get : Outport  Port=3
  wires:
  Switch/1 -> v_cmd/1
  pos_e_feedback/1 -> set_tar_pos when vel_cmd == 0/1(pos_xy_m), Horizontal position controller/2(cur_pos_m)
  set_tar_pos when vel_cmd == 0/1(target_pos_xy_m) -> Cast To Single1/1, Horizontal position controller/1(cur_target_pos_m)
  OR/1 -> delay_on_instant_off/1(in)
  Compare To Constant1/1 -> OR/1
  pos_hold_init/1 -> Unit Delay/1
  Detect Change/1 -> OR/2
  Unit Delay/1 -> Detect Change/1
  Cast To Single1/1 -> Output/1
  ve_y_cmd/1 -> Switch/1, Compare To Constant1/1
  Horizontal position controller/1(ve_xy) -> Mux1/3, Switch/3  "ve_xy"
  NOT/1 -> Switch/2, set_tar_pos when vel_cmd == 0/Enable
  delay_on_instant_off/1(out) -> NOT/1
  Horizontal position controller/3(bearing_to_tar) -> Mux1/2
  Mux1/1 -> Cast To Single/1
  Horizontal position controller/2(dist_to_tar) -> Mux1/1
  Cast To Single/1 -> tar_get/1
  sys/1 -> Horizontal position controller/3(gain)

== system torch_xdof_sim/WAYPOINT CONTROLLER/WP_NAV/Horizontal position controller ==
  Sys_input : Inport
  cur_target_pos_m : Inport  Port=2
  Bus Selector1 : BusSelector  OutputSignals=Sensor Data.tfmini.range_cm
  Cast To Single2 : DataTypeConversion  OutDataTypeStr=single  SaturateOnIntegerOverflow=off  RndMeth=Floor
  Cast To Single3 : DataTypeConversion  OutDataTypeStr=single  SaturateOnIntegerOverflow=off  RndMeth=Floor
  Constant2 : Constant  Value=Aircraft.Control.nav_speed  OutDataTypeStr=single
  Gain : Gain  Gain=0.01
  Ground : Ground
  Horizontal_position_controller : Subsystem
  Mux : Mux  Inputs=2
  Mux1 : Mux  Inputs=3
  "horizontal_error_calculation " : Subsystem
  ve_y_cmd_mps : Outport
  nav_data : Outport  Port=2
  wires:
  Horizontal_position_controller/1(ve_y) -> ve_y_cmd_mps/1
  Sys_input/1 -> Horizontal_position_controller/4(Sys_input), Bus Selector1/1
  "horizontal_error_calculation "/1(dist_to_target_m) -> Horizontal_position_controller/1(dist_to_tar_m), Mux/1
  Bus Selector1/1 -> Mux1/2  "<range_cm>"
  cur_target_pos_m/1 -> "horizontal_error_calculation "/1(target_pos_m)
  Constant2/1 -> Horizontal_position_controller/3(max_v_hor_mps)
  "horizontal_error_calculation "/2(bearing_to_tar_rad) -> Horizontal_position_controller/2(bearing_to_tar_rad), Mux/2
  Mux/1 -> Cast To Single2/1
  Cast To Single2/1 -> nav_data/1
  Ground/1 -> Mux1/1, Mux1/3
  Cast To Single3/1 -> Gain/1
  Gain/1 -> "horizontal_error_calculation "/2(cur_pos_m)  "pos_e_xy"
  Mux1/1 -> Cast To Single3/1

== system torch_xdof_sim/POS_HOLD CONTROLLER/Horizontal speed controller/Subsystem1/roll_D_DLPF ==
  raw_val : Inport
  freq_cut : Inport  Port=2
  Cast To Double1 : DataTypeConversion  OutDataTypeStr=double  SaturateOnIntegerOverflow=off  RndMeth=Floor
  Constant : Constant  Value=50  OutDataTypeStr=single
  MATLAB Function : MATLAB Function  TreatAsAtomicUnit=on
  Unit Delay : UnitDelay  SampleTime=-1  HasFrameUpgradeWarning=on
  filtered_val : Outport
  wires:
  freq_cut/1 -> MATLAB Function/3(freq_cut)
  MATLAB Function/1(filtered_val) -> Unit Delay/1, filtered_val/1
  raw_val/1 -> MATLAB Function/2(raw_val)
  Constant/1 -> MATLAB Function/4(samp_freq)
  Unit Delay/1 -> Cast To Double1/1
  Cast To Double1/1 -> MATLAB Function/1(prev_val)

== system torch_xdof_sim/POS_HOLD CONTROLLER/Horizontal speed controller/zero_vel_handling/Horizontal position controller ==
  cur_target_pos_m : Inport
  cur_pos_m : Inport  Port=2
  gain : Inport  Port=3
  Horizontal_position_controller : Subsystem
  "horizontal_error_calculation " : Subsystem
  ve_xy : Outport
  dist_to_tar : Outport  Port=2
  bearing_to_tar : Outport  Port=3
  wires:
  Horizontal_position_controller/1(Ve_xy) -> ve_xy/1
  "horizontal_error_calculation "/1(dist_to_target_m) -> dist_to_tar/1, Horizontal_position_controller/1(dist_to_tar_m)
  "horizontal_error_calculation "/2(bearing_to_tar_rad) -> bearing_to_tar/1, Horizontal_position_controller/2(direction)
  cur_target_pos_m/1 -> "horizontal_error_calculation "/1(target_pos_m)
  cur_pos_m/1 -> "horizontal_error_calculation "/2(cur_pos_m)
  gain/1 -> Horizontal_position_controller/3(gain)

== system torch_xdof_sim/POS_HOLD CONTROLLER/Horizontal speed controller/zero_vel_handling/delay_on_instant_off ==
  in : Inport
  AND : Logic  IconShape=distinctive  AllPortsSameDT=off  OutDataTypeStr=boolean
  delayed : Subsystem
  out : Outport
  wires:
  delayed/1(delayed_sig) -> AND/1
  in/1 -> AND/2, delayed/1(sig)
  AND/1 -> out/1

== system torch_xdof_sim/POS_HOLD CONTROLLER/Horizontal speed controller/zero_vel_handling/set_tar_pos when vel_cmd == 0 ==
  pos_xy_m : Inport
  Enable : EnablePort
  target_pos_xy_m : Outport
  wires:
  pos_xy_m/1 -> target_pos_xy_m/1
